simulink model "vtolsim"  (R2019a)
settings: Solver=ode45  StartTime=0.0  StopTime=500  RelTol=1e-3  EnableMultiTasking=on
InitFcn:
  | addpath('.')
  | simulation_parameters
values from neighbouring files (symbols this model uses):
  vtol = P    [forces_moments.m]
undefined symbols (not defined in the file or in its folder): drawAircraft, forces_moments, plotvtolstatevariables, u_trim
settings Model: Creator=beard  LastModifiedBy=nikhil
settings DataIOCC: LimitDataPoints=on  SaveFormat=Array  SignalLoggingSaveFormat=ModelDataLogs  ReturnWorkspaceOutputs=off
settings OptimizationCC: ExpressionDepthLimit=2147483647  InitFltsAndDblsToZero=on  LifeSpan=inf
settings DebuggingCC: UnderspecifiedInitializationDetection=Classic  MergeDetectMultiDrivingBlocksExec=none  SolverPrmCheckMsg=warning  FcnCallInpInsideContextMsg=warning  StateNameClashWarn=warning  PregeneratedLibrarySubsystemCodeDiagnostic=none  SFUnexpectedBacktrackingDiag=warning  SFNoUnconditionalDefaultTransitionDiag=warning  SFExecutionAtInitializationDiag=none  ArithmeticOperatorsInVariantConditions=warning
settings HardwareCC: ProdBitPerPointer=32  ProdBitPerSizeT=32  ProdBitPerPtrDiffT=32  ProdLargestAtomicFloat=None  ProdIntDivRoundTo=Undefined  ProdEndianess=Unspecified  ProdWordSize=32  ProdHWDeviceType=32-bit Generic
settings ModelReferenceCC: PropagateSignalLabelsOutOfModel=off
settings SFSimCC: SimUseLocalCustomCode=off
settings RTWCC: RTWUseLocalCustomCode=off
settings CodeAppCC: StateflowObjectComments=on
settings GRTTargetCC: TargetLangStandard=C89/C90 (ANSI)  GeneratePreprocessorConditionals=Disable all  CombineOutputUpdateFcns=off  GRTInterface=on
settings ConfigComp: CovMetricSettings=dw  CovHtmlReporting=on  CovSaveCumulativeToWorkspaceVar=on  CovSaveSingleToWorkspaceVar=on  CovExternalEMLEnable=off  CovSFcnEnable=off

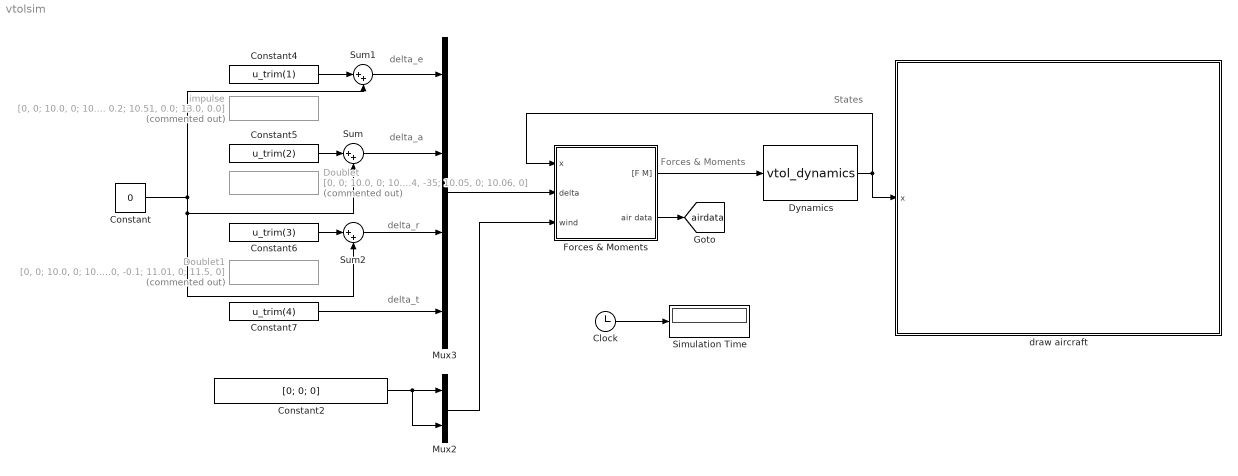
== system vtolsim ==
  note: delta_r
  note: delta_t
  note: Forces & Moments
  note: States
  note: delta_e
  note: delta_a
  Clock : Clock
  Constant : Constant  Value=0
  Constant2 : Constant  Value=[0; 0; 0]
  Constant4 : Constant  Value=u_trim(1)
  Constant5 : Constant  Value=u_trim(2)
  Constant6 : Constant  Value=u_trim(3)
  Constant7 : Constant  Value=u_trim(4)
  Doublet : FromWorkspace  Commented=on  VariableName=[0, 0; 10.0, 0; 10.01, 35; 10.02, 35; 10.03, -35; 10.04, -35; 10.05, 0; 10.06, 0]  SampleTime=0
  Doublet1 : FromWorkspace  Commented=on  VariableName=[0, 0; 10.0, 0; 10.01, 0.1; 10.5, 0.1; 10.51, -0.1; 11.0, -0.1; 11.01, 0; 11.5, 0]  SampleTime=0
  Dynamics : S-Function  FunctionName=vtol_dynamics  Parameters=vtol  SFunctionDeploymentMode=off  EnableBusSupport=off
  Forces & Moments : Subsystem
  Mux2 : Mux  Inputs=2
  Mux3 : Mux
  Simulation Time : Display
  Sum : Sum  Inputs=|++
  Sum1 : Sum  Inputs=|++
  Sum2 : Sum  Inputs=|++
  draw aircraft : Subsystem
      mask Display: image(imread('vtol.jpeg'))
  impulse : FromWorkspace  Commented=on  VariableName=[0, 0; 10.0, 0; 10.01, 0.2; 10.5, 0.2; 10.51, 0.0; 13.0, 0.0]  SampleTime=0
  tag scope: airdata=global
  wires:
  Dynamics/1 -> Forces & Moments/1(x), draw aircraft/1(x)
  Forces & Moments/1("[F M]") -> Dynamics/1
  Clock/1 -> Simulation Time/1
  Forces & Moments/2(air data) -> [airdata]
  Constant2/1 -> Mux2/1, Mux2/2
  Constant5/1 -> Sum/1
  Constant4/1 -> Sum1/1
  Constant6/1 -> Sum2/1
  Mux3/1 -> Forces & Moments/2(delta)
  Mux2/1 -> Forces & Moments/3(wind)
  Sum1/1 -> Mux3/1
  Sum/1 -> Mux3/2
  Sum2/1 -> Mux3/3
  Constant7/1 -> Mux3/4
  Constant/1 -> Sum2/2, Sum/2, Sum1/2

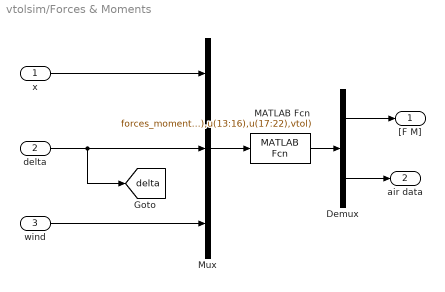
== system vtolsim/Forces & Moments ==
  x : Inport
  delta : Inport  Port=2
  wind : Inport  Port=3
  Demux : Demux  Outputs=[6;6]
  MATLAB Fcn : MATLABFcn  MATLABFcn=forces_moments(u(1:12),u(13:16),u(17:22),vtol)  OutputDimensions=12
  Mux : Mux  Inputs=3
  "[F M]" : Outport
  air data : Outport  Port=2
  tag scope: delta=global
  wires:
  x/1 -> Mux/1
  delta/1 -> [delta], Mux/2
  wind/1 -> Mux/3
  MATLAB Fcn/1 -> Demux/1
  Demux/1 -> "[F M]"/1
  Mux/1 -> MATLAB Fcn/1
  Demux/2 -> air data/1

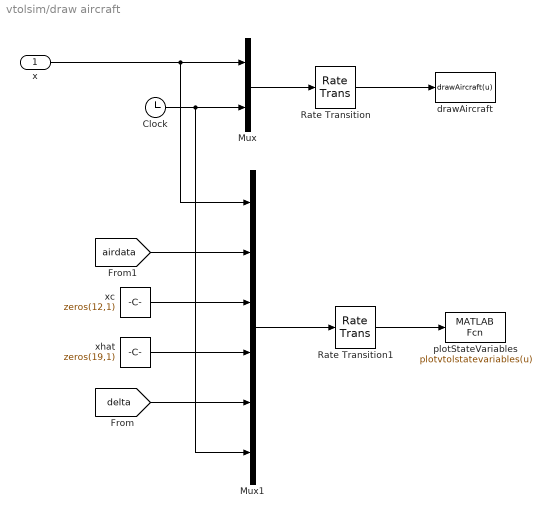
== system vtolsim/draw aircraft ==
  x : Inport
  Clock : Clock
  Mux : Mux  Inputs=2
  Mux1 : Mux  Inputs=6
  Rate Transition : RateTransition  OutPortSampleTimeOpt=Inherit  OutPortSampleTime=SIM.ts_plotting
  Rate Transition1 : RateTransition  OutPortSampleTimeOpt=Inherit  OutPortSampleTime=SIM.ts_plotting
  drawAircraft : MATLABFcn  MATLABFcn=drawAircraft(u)  OutputDimensions=0
  plotStateVariables : MATLABFcn  MATLABFcn=plotvtolstatevariables(u)  OutputDimensions=0
  xc : Constant  Value=zeros(12,1)
  xhat : Constant  Value=zeros(19,1)
  wires:
  [airdata] -> Mux1/2
  [delta] -> Mux1/5
  xc/1 -> Mux1/3
  xhat/1 -> Mux1/4
  Clock/1 -> Mux1/6, Mux/2
  x/1 -> Mux1/1, Mux/1
  Rate Transition1/1 -> plotStateVariables/1
  Mux1/1 -> Rate Transition1/1
  Mux/1 -> Rate Transition/1
  Rate Transition/1 -> drawAircraft/1
